simulink model "TST_EngSpd_DD"  (R2016b)
settings: Solver=FixedStepDiscrete  StartTime=0.0  StopTime=simTime  FixedStep=sampleTime  RelTol=1e-3
values from neighbouring files (symbols this model uses):
  testCase = 1    [initTST_EngSpd_DD_001.m]    (also in initTST_EngSpd_DD_002.m = 2)
libraries: simulink x7, UnitTest_Lib x4
settings Model: Creator=wangzhengfeng  LastModifiedBy=wangzhengfeng
settings DebuggingCC: SignalRangeChecking=error

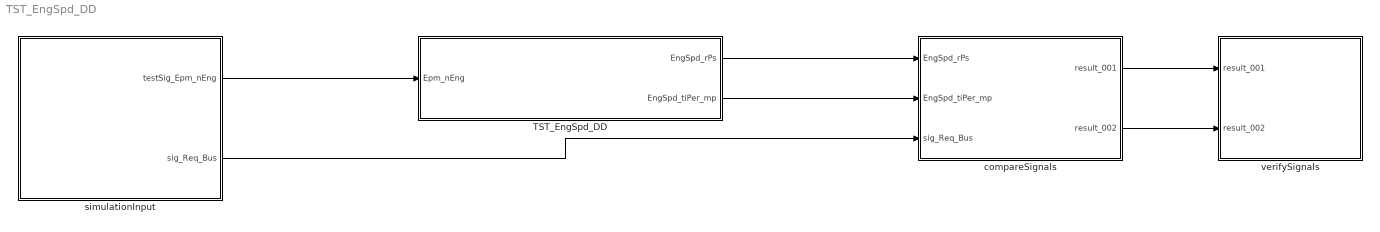
== system TST_EngSpd_DD ==
  TST_EngSpd_DD : Subsystem
  compareSignals : Subsystem
  simulationInput : Subsystem
  verifySignals : Subsystem
  wires:
  simulationInput/1(testSig_Epm_nEng) -> TST_EngSpd_DD/1(Epm_nEng)
  TST_EngSpd_DD/1(EngSpd_rPs) -> compareSignals/1(EngSpd_rPs)
  TST_EngSpd_DD/2(EngSpd_tiPer_mp) -> compareSignals/2(EngSpd_tiPer_mp)
  simulationInput/2(sig_Req_Bus) -> compareSignals/3(sig_Req_Bus)
  compareSignals/1(result_001) -> verifySignals/1(result_001)
  compareSignals/2(result_002) -> verifySignals/2(result_002)

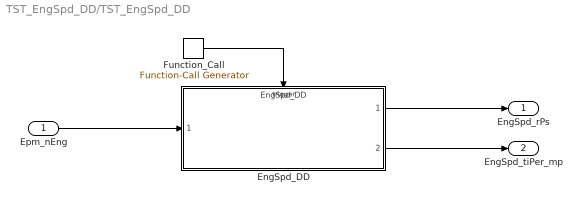
== system TST_EngSpd_DD/TST_EngSpd_DD ==
  Epm_nEng : Inport
  EngSpd_DD : ModelReference  ModelNameDialog=EngSpd_DD  SimulationMode=Normal  ModelReferenceVersion=1.23  TriggerPortName=function  TriggerPortTriggerType=function-call  TriggerPortStatesWhenEnabling=held
  Function_Call : simulink/Ports & Subsystems/Function-Call Generator  sample_time=sampleTime  numberOfIterations=1
  EngSpd_rPs : Outport
  EngSpd_tiPer_mp : Outport  Port=2
  wires:
  Function_Call/1 -> EngSpd_DD/Trigger
  Epm_nEng/1 -> EngSpd_DD/1
  EngSpd_DD/1 -> EngSpd_rPs/1
  EngSpd_DD/2 -> EngSpd_tiPer_mp/1

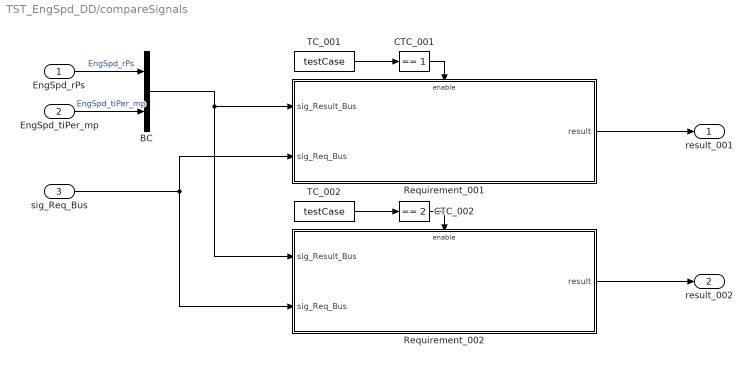
== system TST_EngSpd_DD/compareSignals ==
  EngSpd_rPs : Inport
  EngSpd_tiPer_mp : Inport  Port=2
  sig_Req_Bus : Inport  Port=3
  BC : BusCreator  Inputs=2
  CTC_001 : simulink/Logic and Bit Operations/Compare To Constant  relop===  const=1  OutDataTypeStr=boolean
  CTC_002 : simulink/Logic and Bit Operations/Compare To Constant  relop===  const=2  OutDataTypeStr=boolean
  Requirement_001 : Subsystem
  Requirement_002 : Subsystem
  TC_001 : Constant  Value=testCase
  TC_002 : Constant  Value=testCase
  result_001 : Outport
  result_002 : Outport  Port=2
  wires:
  EngSpd_rPs/1 -> BC/1  "EngSpd_rPs"
  EngSpd_tiPer_mp/1 -> BC/2  "EngSpd_tiPer_mp"
  TC_001/1 -> CTC_001/1
  CTC_001/1 -> Requirement_001/Enable
  sig_Req_Bus/1 -> Requirement_001/2(sig_Req_Bus), Requirement_002/2(sig_Req_Bus)
  BC/1 -> Requirement_001/1(sig_Result_Bus), Requirement_002/1(sig_Result_Bus)
  Requirement_001/1(result) -> result_001/1
  TC_002/1 -> CTC_002/1
  CTC_002/1 -> Requirement_002/Enable
  Requirement_002/1(result) -> result_002/1

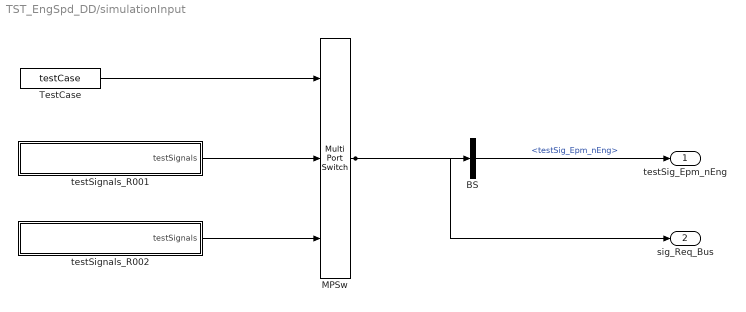
== system TST_EngSpd_DD/simulationInput ==
  BS : BusSelector  OutputSignals=testSig_Epm_nEng
  MPSw : MultiPortSwitch  Inputs=2  SaturateOnIntegerOverflow=on  InputSameDT=on
  TestCase : Constant  Value=testCase
  testSignals_R001 : Subsystem
  testSignals_R002 : Subsystem
  testSig_Epm_nEng : Outport
  sig_Req_Bus : Outport  Port=2
  wires:
  BS/1 -> testSig_Epm_nEng/1  "<testSig_Epm_nEng>"
  MPSw/1 -> BS/1, sig_Req_Bus/1
  TestCase/1 -> MPSw/1
  testSignals_R001/1(testSignals) -> MPSw/2
  testSignals_R002/1(testSignals) -> MPSw/3

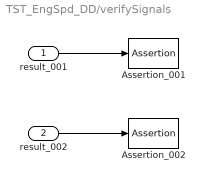
== system TST_EngSpd_DD/verifySignals ==
  result_001 : Inport
  result_002 : Inport  Port=2
  Assertion_001 : Assertion  Enabled=off
  Assertion_002 : Assertion  Enabled=off
  wires:
  result_001/1 -> Assertion_001/1
  result_002/1 -> Assertion_002/1

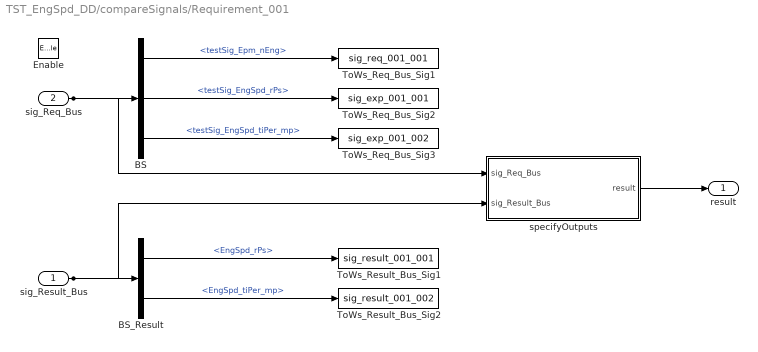
== system TST_EngSpd_DD/compareSignals/Requirement_001 ==
  sig_Result_Bus : Inport
  sig_Req_Bus : Inport  Port=2
  Enable : EnablePort
  BS : BusSelector  OutputSignals=testSig_Epm_nEng,testSig_EngSpd_rPs,testSig_EngSpd_tiPer_mp
  BS_Result : BusSelector  OutputSignals=EngSpd_rPs,EngSpd_tiPer_mp
  ToWs_Req_Bus_Sig1 : ToWorkspace  VariableName=sig_req_001_001  SaveFormat=Structure With Time
  ToWs_Req_Bus_Sig2 : ToWorkspace  VariableName=sig_exp_001_001  SaveFormat=Structure With Time
  ToWs_Req_Bus_Sig3 : ToWorkspace  VariableName=sig_exp_001_002  SaveFormat=Structure With Time
  ToWs_Result_Bus_Sig1 : ToWorkspace  VariableName=sig_result_001_001  SaveFormat=Structure With Time
  ToWs_Result_Bus_Sig2 : ToWorkspace  VariableName=sig_result_001_002  SaveFormat=Structure With Time
  specifyOutputs : Subsystem
  result : Outport
  wires:
  sig_Req_Bus/1 -> BS/1, specifyOutputs/1(sig_Req_Bus)
  BS/1 -> ToWs_Req_Bus_Sig1/1  "<testSig_Epm_nEng>"
  BS/2 -> ToWs_Req_Bus_Sig2/1  "<testSig_EngSpd_rPs>"
  BS/3 -> ToWs_Req_Bus_Sig3/1  "<testSig_EngSpd_tiPer_mp>"
  sig_Result_Bus/1 -> BS_Result/1, specifyOutputs/2(sig_Result_Bus)
  BS_Result/1 -> ToWs_Result_Bus_Sig1/1  "<EngSpd_rPs>"
  BS_Result/2 -> ToWs_Result_Bus_Sig2/1  "<EngSpd_tiPer_mp>"
  specifyOutputs/1(result) -> result/1

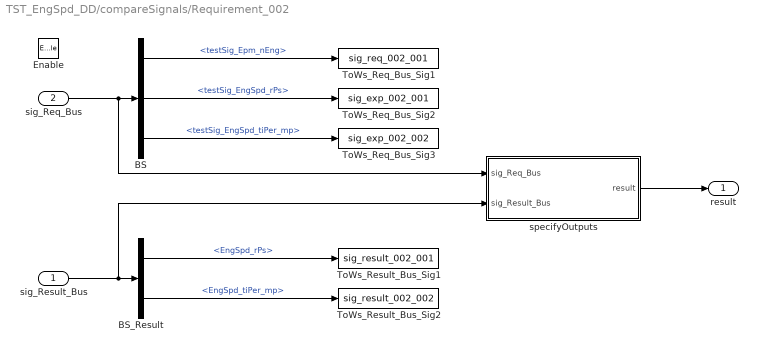
== system TST_EngSpd_DD/compareSignals/Requirement_002 ==
  sig_Result_Bus : Inport
  sig_Req_Bus : Inport  Port=2
  Enable : EnablePort
  BS : BusSelector  OutputSignals=testSig_Epm_nEng,testSig_EngSpd_rPs,testSig_EngSpd_tiPer_mp
  BS_Result : BusSelector  OutputSignals=EngSpd_rPs,EngSpd_tiPer_mp
  ToWs_Req_Bus_Sig1 : ToWorkspace  VariableName=sig_req_002_001  SaveFormat=Structure With Time
  ToWs_Req_Bus_Sig2 : ToWorkspace  VariableName=sig_exp_002_001  SaveFormat=Structure With Time
  ToWs_Req_Bus_Sig3 : ToWorkspace  VariableName=sig_exp_002_002  SaveFormat=Structure With Time
  ToWs_Result_Bus_Sig1 : ToWorkspace  VariableName=sig_result_002_001  SaveFormat=Structure With Time
  ToWs_Result_Bus_Sig2 : ToWorkspace  VariableName=sig_result_002_002  SaveFormat=Structure With Time
  specifyOutputs : Subsystem
  result : Outport
  wires:
  sig_Req_Bus/1 -> BS/1, specifyOutputs/1(sig_Req_Bus)
  BS/1 -> ToWs_Req_Bus_Sig1/1  "<testSig_Epm_nEng>"
  BS/2 -> ToWs_Req_Bus_Sig2/1  "<testSig_EngSpd_rPs>"
  BS/3 -> ToWs_Req_Bus_Sig3/1  "<testSig_EngSpd_tiPer_mp>"
  sig_Result_Bus/1 -> BS_Result/1, specifyOutputs/2(sig_Result_Bus)
  BS_Result/1 -> ToWs_Result_Bus_Sig1/1  "<EngSpd_rPs>"
  BS_Result/2 -> ToWs_Result_Bus_Sig2/1  "<EngSpd_tiPer_mp>"
  specifyOutputs/1(result) -> result/1

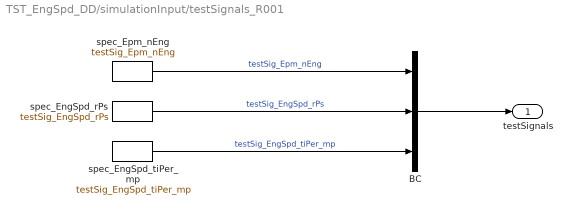
== system TST_EngSpd_DD/simulationInput/testSignals_R001 ==
  BC : BusCreator  Inputs=3
  spec_EngSpd_rPs : FromWorkspace  VariableName=testSig_EngSpd_rPs  Interpolate=off  OutputAfterFinalValue=Holding final value
  spec_EngSpd_tiPer_mp : FromWorkspace  VariableName=testSig_EngSpd_tiPer_mp  Interpolate=off  OutputAfterFinalValue=Holding final value
  spec_Epm_nEng : FromWorkspace  VariableName=testSig_Epm_nEng  Interpolate=off  OutputAfterFinalValue=Holding final value
  testSignals : Outport
  wires:
  BC/1 -> testSignals/1
  spec_Epm_nEng/1 -> BC/1  "testSig_Epm_nEng"
  spec_EngSpd_rPs/1 -> BC/2  "testSig_EngSpd_rPs"
  spec_EngSpd_tiPer_mp/1 -> BC/3  "testSig_EngSpd_tiPer_mp"

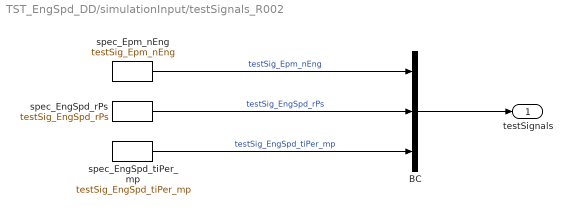
== system TST_EngSpd_DD/simulationInput/testSignals_R002 ==
  BC : BusCreator  Inputs=3
  spec_EngSpd_rPs : FromWorkspace  VariableName=testSig_EngSpd_rPs  Interpolate=off  OutputAfterFinalValue=Holding final value
  spec_EngSpd_tiPer_mp : FromWorkspace  VariableName=testSig_EngSpd_tiPer_mp  Interpolate=off  OutputAfterFinalValue=Holding final value
  spec_Epm_nEng : FromWorkspace  VariableName=testSig_Epm_nEng  Interpolate=off  OutputAfterFinalValue=Holding final value
  testSignals : Outport
  wires:
  BC/1 -> testSignals/1
  spec_Epm_nEng/1 -> BC/1  "testSig_Epm_nEng"
  spec_EngSpd_rPs/1 -> BC/2  "testSig_EngSpd_rPs"
  spec_EngSpd_tiPer_mp/1 -> BC/3  "testSig_EngSpd_tiPer_mp"

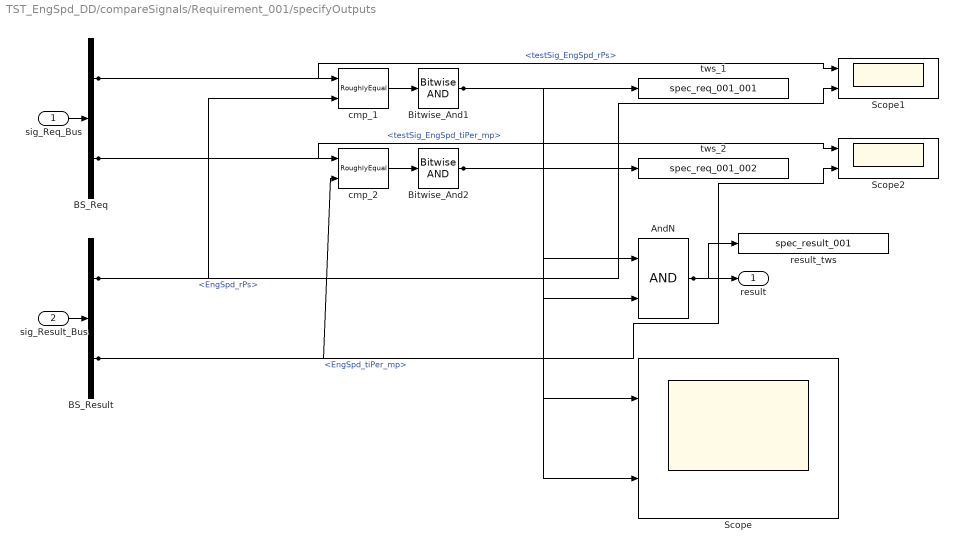
== system TST_EngSpd_DD/compareSignals/Requirement_001/specifyOutputs ==
  sig_Req_Bus : Inport
  sig_Result_Bus : Inport  Port=2
  AndN : Logic
  BS_Req : BusSelector  OutputSignals=testSig_EngSpd_rPs,testSig_EngSpd_tiPer_mp
  BS_Result : BusSelector  OutputSignals=EngSpd_rPs,EngSpd_tiPer_mp
  Bitwise_And1 : simulink/Logic and Bit Operations/Bitwise Operator  logicop=AND  UseBitMask=off  BitMask=bin2dec('11011001')  BitMaskRealWorld=Stored Integer
  Bitwise_And2 : simulink/Logic and Bit Operations/Bitwise Operator  logicop=AND  UseBitMask=off  BitMask=bin2dec('11011001')  BitMaskRealWorld=Stored Integer
  Scope : Scope  NumInputPorts=2
  Scope1 : Scope  NumInputPorts=2
  Scope2 : Scope  NumInputPorts=2
  cmp_1 : UnitTest_Lib/RoughlyEqual  slope=0.1
  cmp_2 : UnitTest_Lib/RoughlyEqual  slope=0.1
  result_tws : ToWorkspace  VariableName=spec_result_001
  tws_1 : ToWorkspace  VariableName=spec_req_001_001
  tws_2 : ToWorkspace  VariableName=spec_req_001_002
  result : Outport
  wires:
  sig_Req_Bus/1 -> BS_Req/1
  sig_Result_Bus/1 -> BS_Result/1
  AndN/1 -> result/1, result_tws/1
  BS_Req/1 -> cmp_1/1, Scope1/1  "<testSig_EngSpd_rPs>"
  BS_Result/1 -> cmp_1/2, Scope1/2  "<EngSpd_rPs>"
  cmp_1/1 -> Bitwise_And1/1
  Bitwise_And1/1 -> tws_1/1, AndN/1, Scope/1
  BS_Req/2 -> cmp_2/1, Scope2/1  "<testSig_EngSpd_tiPer_mp>"
  BS_Result/2 -> cmp_2/2, Scope2/2  "<EngSpd_tiPer_mp>"
  cmp_2/1 -> Bitwise_And2/1
  Bitwise_And2/1 -> tws_2/1, AndN/2, Scope/2

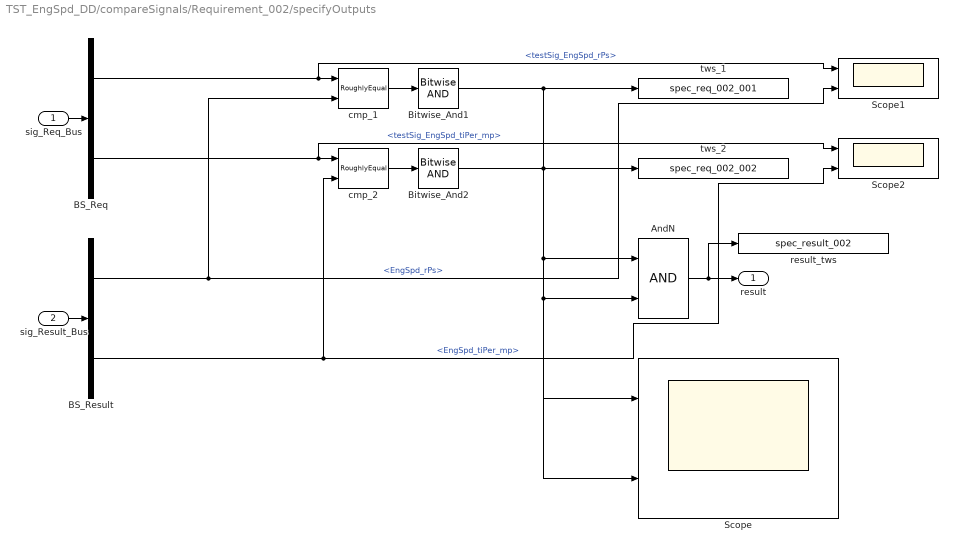
== system TST_EngSpd_DD/compareSignals/Requirement_002/specifyOutputs ==
  sig_Req_Bus : Inport
  sig_Result_Bus : Inport  Port=2
  AndN : Logic
  BS_Req : BusSelector  OutputSignals=testSig_EngSpd_rPs,testSig_EngSpd_tiPer_mp
  BS_Result : BusSelector  OutputSignals=EngSpd_rPs,EngSpd_tiPer_mp
  Bitwise_And1 : simulink/Logic and Bit Operations/Bitwise Operator  logicop=AND  UseBitMask=off  BitMask=bin2dec('11011001')  BitMaskRealWorld=Stored Integer
  Bitwise_And2 : simulink/Logic and Bit Operations/Bitwise Operator  logicop=AND  UseBitMask=off  BitMask=bin2dec('11011001')  BitMaskRealWorld=Stored Integer
  Scope : Scope  NumInputPorts=2
  Scope1 : Scope  NumInputPorts=2
  Scope2 : Scope  NumInputPorts=2
  cmp_1 : UnitTest_Lib/RoughlyEqual  slope=0.1
  cmp_2 : UnitTest_Lib/RoughlyEqual  slope=0.1
  result_tws : ToWorkspace  VariableName=spec_result_002
  tws_1 : ToWorkspace  VariableName=spec_req_002_001
  tws_2 : ToWorkspace  VariableName=spec_req_002_002
  result : Outport
  wires:
  sig_Req_Bus/1 -> BS_Req/1
  sig_Result_Bus/1 -> BS_Result/1
  AndN/1 -> result/1, result_tws/1
  BS_Req/1 -> cmp_1/1, Scope1/1  "<testSig_EngSpd_rPs>"
  BS_Result/1 -> cmp_1/2, Scope1/2  "<EngSpd_rPs>"
  cmp_1/1 -> Bitwise_And1/1
  Bitwise_And1/1 -> AndN/1, Scope/1, tws_1/1
  BS_Req/2 -> cmp_2/1, Scope2/1  "<testSig_EngSpd_tiPer_mp>"
  BS_Result/2 -> cmp_2/2, Scope2/2  "<EngSpd_tiPer_mp>"
  cmp_2/1 -> Bitwise_And2/1
  Bitwise_And2/1 -> AndN/2, Scope/2, tws_2/1
